simulink model "w1p5"  (R2020a)
settings: Solver=VariableStepAuto  StartTime=0.0  StopTime=10  RelTol=1e-3
values from neighbouring files (symbols this model uses):
  C = 1e-05    [w1p5.mat]
  R = 10    [w1p5.mat]
libraries: simulink x2
settings Model: Creator=Shubham  LastModifiedBy=Shubham

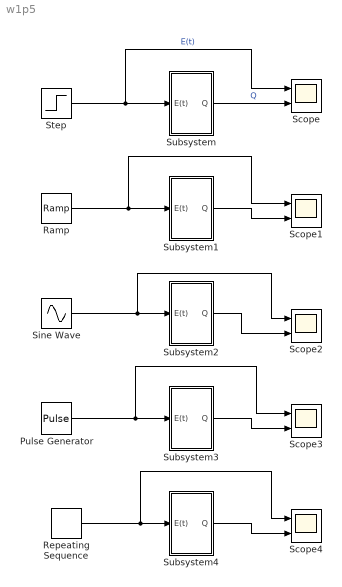
== system w1p5 ==
  Pulse Generator : DiscretePulseGenerator  PulseType=Time based  Period=10  PulseWidth=5
  Ramp : simulink/Sources/Ramp  slope=1  start=0  InitialOutput=0
  Repeating Sequence : simulink/Sources/Repeating Sequence  rep_seq_t=[0 2]  rep_seq_y=[0 2]
  Scope{,1..4} (5 alike) : Scope  NumInputPorts=2
  Sine Wave : Sin  SampleTime=0
  Step : Step  After=5  SampleTime=0
  Subsystem : Subsystem
  Subsystem1 : Subsystem
  Subsystem2 : Subsystem
  Subsystem3 : Subsystem
  Subsystem4 : Subsystem
  wires:
  Step/1 -> Scope/1, Subsystem/1(E(t))  "E(t)"
  Subsystem/1(Q) -> Scope/2  "Q"
  Ramp/1 -> Scope1/1, Subsystem1/1(E(t))
  Subsystem1/1(Q) -> Scope1/2
  Subsystem2/1(Q) -> Scope2/2
  Subsystem3/1(Q) -> Scope3/2
  Subsystem4/1(Q) -> Scope4/2
  Sine Wave/1 -> Scope2/1, Subsystem2/1(E(t))
  Pulse Generator/1 -> Scope3/1, Subsystem3/1(E(t))
  Repeating Sequence/1 -> Scope4/1, Subsystem4/1(E(t))

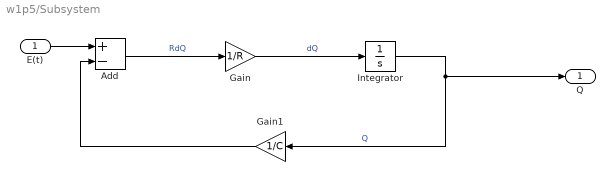
== system w1p5/Subsystem ==
  E(t) : Inport
  Add : Sum  Inputs=+-
  Gain : Gain  Gain=1/R
  Gain1 : Gain  Gain=1/C
  Integrator : Integrator
  Q : Outport
  wires:
  Add/1 -> Gain/1  "RdQ"
  Integrator/1 -> Q/1, Gain1/1  "Q"
  Gain/1 -> Integrator/1  "dQ"
  Gain1/1 -> Add/2
  E(t)/1 -> Add/1

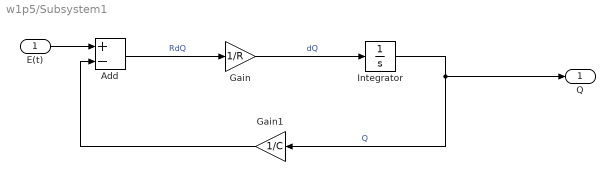
== system w1p5/Subsystem1 ==
  E(t) : Inport
  Add : Sum  Inputs=+-
  Gain : Gain  Gain=1/R
  Gain1 : Gain  Gain=1/C
  Integrator : Integrator  InitialCondition=1
  Q : Outport
  wires:
  Add/1 -> Gain/1  "RdQ"
  Integrator/1 -> Q/1, Gain1/1  "Q"
  Gain/1 -> Integrator/1  "dQ"
  Gain1/1 -> Add/2
  E(t)/1 -> Add/1

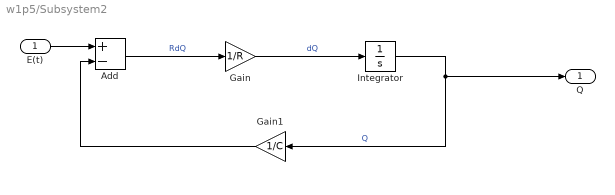
== system w1p5/Subsystem2 ==
  E(t) : Inport
  Add : Sum  Inputs=+-
  Gain : Gain  Gain=1/R
  Gain1 : Gain  Gain=1/C
  Integrator : Integrator  InitialCondition=0.2
  Q : Outport
  wires:
  Add/1 -> Gain/1  "RdQ"
  Integrator/1 -> Q/1, Gain1/1  "Q"
  Gain/1 -> Integrator/1  "dQ"
  Gain1/1 -> Add/2
  E(t)/1 -> Add/1

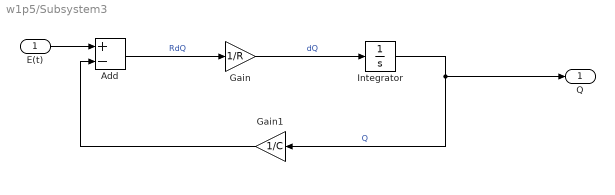
== system w1p5/Subsystem3 ==
  E(t) : Inport
  Add : Sum  Inputs=+-
  Gain : Gain  Gain=1/R
  Gain1 : Gain  Gain=1/C
  Integrator : Integrator  InitialCondition=0.5
  Q : Outport
  wires:
  Add/1 -> Gain/1  "RdQ"
  Integrator/1 -> Q/1, Gain1/1  "Q"
  Gain/1 -> Integrator/1  "dQ"
  Gain1/1 -> Add/2
  E(t)/1 -> Add/1

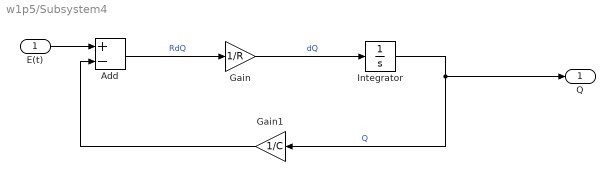
== system w1p5/Subsystem4 ==
  E(t) : Inport
  Add : Sum  Inputs=+-
  Gain : Gain  Gain=1/R
  Gain1 : Gain  Gain=1/C
  Integrator : Integrator  InitialCondition=0.8
  Q : Outport
  wires:
  Add/1 -> Gain/1  "RdQ"
  Integrator/1 -> Q/1, Gain1/1  "Q"
  Gain/1 -> Integrator/1  "dQ"
  Gain1/1 -> Add/2
  E(t)/1 -> Add/1
